simulink model "workload"  (Simulink 5.0)
settings: Solver=ode1  StartTime=0.0  StopTime=TIME_SFT(end)  FixedStep=0.02  RelTol=1e-3
settings Model: LastModifiedBy=E183308

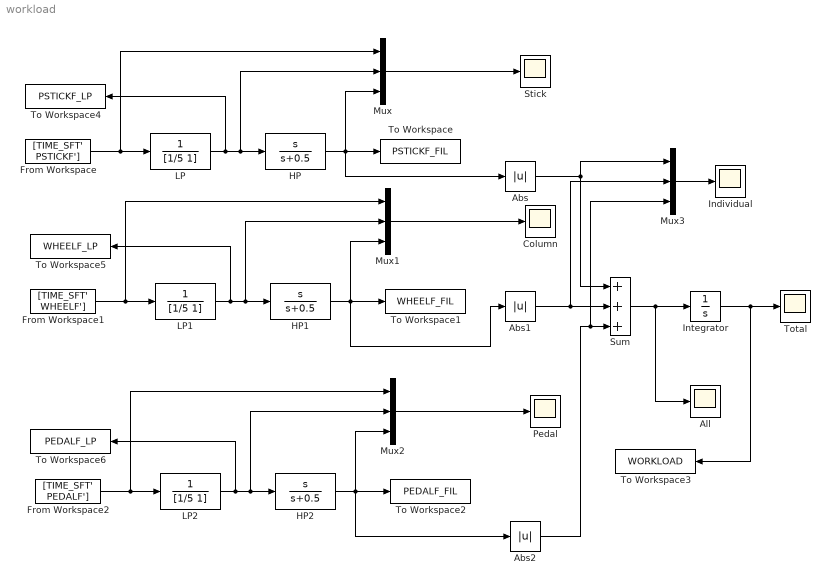
== system workload ==
  Abs : Abs  SaturateOnIntegerOverflow=on
  Abs1 : Abs  SaturateOnIntegerOverflow=on
  Abs2 : Abs  SaturateOnIntegerOverflow=on
  All : Scope
      settings: SaveName=ScopeData5
  Column : Scope
  From Workspace : FromWorkspace  VariableName=[TIME_SFT' PSTICKF']  SampleTime=0
  From Workspace1 : FromWorkspace  VariableName=[TIME_SFT' WHEELF']  SampleTime=0
  From Workspace2 : FromWorkspace  VariableName=[TIME_SFT' PEDALF']  SampleTime=0
  HP : TransferFcn  Numerator=[1 0]  Denominator=[1 0.5]
  HP1 : TransferFcn  Numerator=[1 0]  Denominator=[1 0.5]
  HP2 : TransferFcn  Numerator=[1 0]  Denominator=[1 0.5]
  Individual : Scope
      settings: SaveName=ScopeData4
  Integrator : Integrator
  LP : TransferFcn  Denominator=[1/5 1]
  LP1 : TransferFcn  Denominator=[1/5 1]
  LP2 : TransferFcn  Denominator=[1/5 1]
  Mux{,1..3} (4 alike) : Mux  Inputs=3
  Pedal : Scope
      settings: SaveName=ScopeData2
  Stick : Scope
  Sum : Sum  Inputs=+++  SaturateOnIntegerOverflow=on
  To Workspace : ToWorkspace  VariableName=PSTICKF_FIL  SampleTime=-1  SaveFormat=Array
  To Workspace1 : ToWorkspace  VariableName=WHEELF_FIL  SampleTime=-1  SaveFormat=Array
  To Workspace2 : ToWorkspace  VariableName=PEDALF_FIL  SampleTime=-1  SaveFormat=Array
  To Workspace3 : ToWorkspace  VariableName=WORKLOAD  SampleTime=-1  SaveFormat=Array
  To Workspace4 : ToWorkspace  VariableName=PSTICKF_LP  SampleTime=-1  SaveFormat=Array
  To Workspace5 : ToWorkspace  VariableName=WHEELF_LP  SampleTime=-1  SaveFormat=Array
  To Workspace6 : ToWorkspace  VariableName=PEDALF_LP  SampleTime=-1  SaveFormat=Array
  Total : Scope
      settings: SaveName=ScopeData3
  wires:
  From Workspace/1 -> LP/1, Mux/1
  LP/1 -> HP/1, Mux/2, To Workspace4/1
  HP/1 -> To Workspace/1, Mux/3, Abs/1
  Mux/1 -> Stick/1
  From Workspace1/1 -> LP1/1, Mux1/1
  LP1/1 -> HP1/1, Mux1/2, To Workspace5/1
  HP1/1 -> To Workspace1/1, Mux1/3, Abs1/1
  Mux1/1 -> Column/1
  From Workspace2/1 -> LP2/1, Mux2/1
  LP2/1 -> HP2/1, Mux2/2, To Workspace6/1
  HP2/1 -> To Workspace2/1, Mux2/3, Abs2/1
  Mux2/1 -> Pedal/1
  Sum/1 -> Integrator/1, All/1
  Mux3/1 -> Individual/1
  Integrator/1 -> Total/1, To Workspace3/1
  Abs/1 -> Sum/1, Mux3/1
  Abs1/1 -> Sum/2, Mux3/2
  Abs2/1 -> Sum/3, Mux3/3
